simulink model "Electrolyzer"  (R2024b)
settings: Solver=VariableStepAuto  StartTime=0.0  StopTime=3600  RelTol=1e-3
undefined symbols (not defined in the file or in its folder): DiscIntNeverNeededParam
libraries: nesl_utility x9, fl_lib x2, ee_lib x1
settings Model: LastModifiedBy=razpo

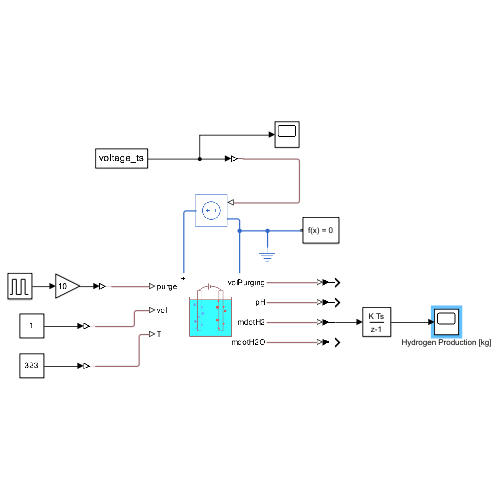
[thumbnail: Simulink's stored preview of the top-level diagram]
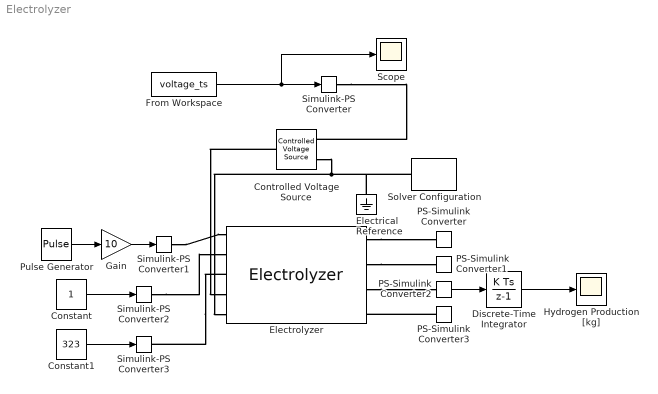
== system Electrolyzer ==
  Constant : Constant
  Constant1 : Constant  Value=323
  Controlled Voltage Source : fl_lib/Electrical/Electrical Sources/Controlled Voltage Source
  Discrete-Time Integrator : DiscreteIntegrator  gainval=1/3600  SampleTime=10  ICPrevOutput=DiscIntNeverNeededParam  ICPrevScaledInput=DiscIntNeverNeededParam
  Electrical Reference : fl_lib/Electrical/Electrical Elements/Electrical Reference
  Electrolyzer : ee_lib/Sources/Electrolyzer  pH_option=ee.enum.electrolyzer.pH.constant  R=0.25 Ohm  area=30000 cm^2  x=2 cm  NCells=100  pH0=7  pHC=6  pH_vec=[5, 5.5, 6, 6.5, 7]  rho_vec=[.2, .75, 2.5, 8, 18.2] MOhm*cm  T_vec=[273, 298, 323, 348, 373] K  eff_vec=ones(5, 1)  i_specify=off  i_priority=None  i=0 A  i_nominal_specify=off  i_nominal_value=1  i_nominal_unit=A  v_specify=off  v_priority=None  v=100 V  v_nominal_specify=off  v_nominal_value=100  v_nominal_unit=V  PE_specify=off  PE_priority=None  PE=100 J/s  PE_nominal_specify=off  PE_nominal_value=1  PE_nominal_unit=J/s  mol_e_specify=off  mol_e_priority=None  mol_e=1e3 mol/s  mol_e_nominal_specify=off  mol_e_nominal_value=1  mol_e_nominal_unit=mol/s  mol_h2_specify=off  mol_h2_priority=None  mol_h2=1e3 mol/s  mol_h2_nominal_specify=off  mol_h2_nominal_value=1  mol_h2_nominal_unit=mol/s  RT_specify=off  RT_priority=None  RT=1 Ohm  RT_nominal_specify=off  RT_nominal_value=1  RT_nominal_unit=Ohm  xhp_specify=off  xhp_priority=None  xhp=1 mol  xhp_nominal_specify=off  xhp_nominal_value=1  xhp_nominal_unit=mol
      settings: InternalSimscapePortConfiguration="{\"Bottom\":[],\"Left\":[{\"id\":\"purge\",\"label\":\"purge\",\"type\":\"input\"},{\"id\":\"vol\",\"label\":\"vol\",\"type\":\"input\"},{\"id\":\"T\",\"label\":\"T\",\"type\":\"input\"}],\"Right\":[{\"id\":\"volPurging\",\"label\":\"volPurging\",\"type\":\"output\"},{\"id\":\"pH\",\"label\":\"pH\",\"type\":\"output\"},{\"id\":\"mdotH2\",\"label\":\"mdotH2\",\"type\":\"output\"},{\"id\":\"mdotH2O\",\"label\":\"mdotH2O\",\"type\":\"output\"}],\"Top\":[{\"id\":\"p\",\"label\":\"+\",\"type\":\"foundation.electrical.electrical\"},{\"id\":\"n\",\"label\":\"-\",\"type\":\"foundation.electrical.electrical\"}]}"
  From Workspace : FromWorkspace  VariableName=voltage_ts
  Gain : Gain  Gain=10
  Hydrogen Production [kg] : Scope
  PS-Simulink Converter{,1..3} (4 alike) : nesl_utility/PS-Simulink Converter  PhysicalDomain=network_engine_domain  SubClassName=ps_output  LeftPortType=input  RightPortType=output  PseudoPeriodic=off  Frequencies=[]  VectorFormat=inherit  Unit=inherit  AffineConversion=off
  Pulse Generator : DiscretePulseGenerator  PulseType=Time based  Period=10  PulseWidth=5
  Scope : Scope
  Simulink-PS Converter{,1..3} (4 alike) : nesl_utility/Simulink-PS Converter  PhysicalDomain=network_engine_domain  SubClassName=ps_input  LeftPortType=input  RightPortType=output  PseudoPeriodic=off  Frequencies=[]  NoiseDistribution=none  NoiseParameters=[]  Unit=1  AffineConversion=off  FilteringAndDerivatives=provide  SimscapeFilterOrder=1  InputFilterTimeConstant=0.001  UdotUserProvided=0
  Solver Configuration : nesl_utility/Solver Configuration  PhysicalDomain=network_engine_domain  SubClassName=solver  LeftPortType=input  RightPortType=generic  Tones=[]  Harmonics=[]  SimulateNoise=off  Profile=off  UseLocalSampling=off  EnableSwitchedLinearOptims=on  FrequencyDomain=off  UseCCode=off  RelTol=0.001  AbsTol=0.001  MinStep=1e-09  ToWorkspace=off  RevertToSquareIcSolve=off  NumHomotopyIterations=100  PhasorMode=off  PhasorModeNumHarmonics=1  ConsistencySolver=NEWTON_XTOL_AFTER_FTOL  IndexReductionMethod=DerivativeReplacement  DoDC=off  ResidualTolerance=1e-09  ConsistencyTolSource=GLOBAL  ConsistencyAbsTol=0.001  ConsistencyRelTol=0.001  ConsistencyTolFactor=0.001  UseLocalSolver=off  LocalSolverChoice=NE_BACKWARD_EULER_ADVANCER  ResolveIndetEquations=on  FunctionEvalNumThread=1  LocalSolverSampleTime=0.001  DoFixedCost=off  MaxNonlinIter=3  MaxModeIter=2  ComputeImpulses=off  ImpulseIterations=2  LinearAlgebra=auto  LinearAlgebraNumThread=0  EquationFormulation=NE_TIME_EF  DelaysMemoryBudget=1024  AutomaticFiltering=on  FilteringTimeConstant=0.001  PartitionStorageMethod=AS_NEEDED  PartitionMemoryBudget=1024  PartitionMethod=ROBUST  MultibodyUseLocalSolver=off  MultibodyLocalSolverChoice=ODE1  MultibodyLocalSolverSampleTime=0.001
  wires:
  From Workspace/1 -> Scope/1, Simulink-PS Converter/1
  Pulse Generator/1 -> Gain/1
  Constant/1 -> Simulink-PS Converter2/1
  Constant1/1 -> Simulink-PS Converter3/1
  Gain/1 -> Simulink-PS Converter1/1
  PS-Simulink Converter2/1 -> Discrete-Time Integrator/1
  Discrete-Time Integrator/1 -> Hydrogen Production [kg]/1
  connections:
  Simulink-PS Converter/RConn1 -- Controlled Voltage Source/RConn1
  Controlled Voltage Source/RConn2 -- Electrical Reference/LConn1 -- Solver Configuration/RConn1 -- Electrolyzer/LConn5
  Simulink-PS Converter1/RConn1 -- Electrolyzer/LConn1
  Simulink-PS Converter2/RConn1 -- Electrolyzer/LConn2
  Electrolyzer/LConn3 -- Simulink-PS Converter3/RConn1
  Electrolyzer/RConn1 -- PS-Simulink Converter/LConn1
  Electrolyzer/RConn2 -- PS-Simulink Converter1/LConn1
  PS-Simulink Converter3/LConn1 -- Electrolyzer/RConn4
  Controlled Voltage Source/LConn1 -- Electrolyzer/LConn4
  Electrolyzer/RConn3 -- PS-Simulink Converter2/LConn1
